simulink model "TwoTankS11_Owen_v6"  (Simulink 9.1)
settings: Solver=ode3  StartTime=0.0  StopTime=999  FixedStep=1/10  RelTol=1e-3  EnableMultiTasking=on
undefined symbols (not defined in the file or in its folder): MIO, National_Instruments, PCI
libraries: sldrtlib x3
settings Model: Creator=fowen  LastModifiedBy=melab2  SimulationMode=external  ExtModeTrigDuration=10000
settings DataIOCC: LimitDataPoints=on  MaxDataPoints=100000  SignalLoggingSaveFormat=ModelDataLogs
settings OptimizationCC: ExpressionDepthLimit=2147483647  LifeSpan=auto
settings DebuggingCC: SolverPrmCheckMsg=warning  FcnCallInpInsideContextMsg=warning  StateNameClashWarn=warning
settings HardwareCC: ProdBitPerPointer=64  ProdBitPerSizeT=64  ProdBitPerPtrDiffT=64  ProdLargestAtomicFloat=Float  ProdIntDivRoundTo=Zero  ProdEndianess=LittleEndian  ProdWordSize=64  ProdHWDeviceType=Intel->x86-64 (Windows64)
settings RTWCC: SystemTargetFile=sldrt.tlc  TemplateMakefile=sldrt.tmf  Description=Simulink Desktop Real-Time  RTWCompilerOptimization=on
settings CodeAppCC: MaxIdLength=95
settings SimulinkDesktopRealTimeCC: TargetPreCompLibLocation=C:\Program Files\MATLAB\R2018a\toolbox\sldrt\lib\win64  TargetLangStandard=C89/C90 (ANSI)  SupportVariableSizeSignals=off
settings ConfigComp: CovSFcnEnable=off

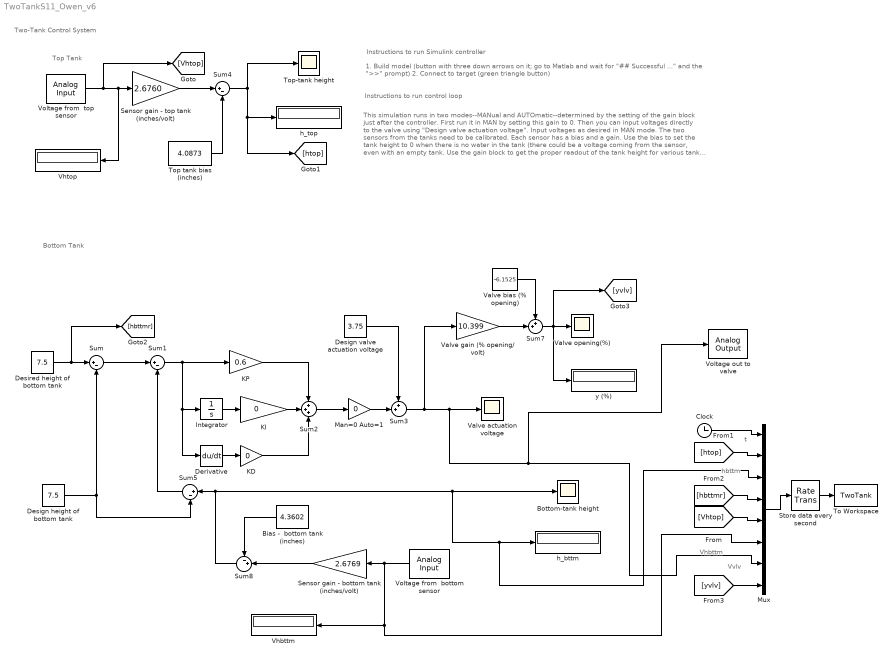
== system TwoTankS11_Owen_v6 ==
  note: Two-Tank Control System
  note: Top Tank
  note: Vhbttm
  note: Vvlv
  note: hbttm
  note: This simulation runs in two modes--MANual and AUTOmatic--determined by the setting of the gain block just after
      | the controller.  First run it in MAN by setting this gain to 0.  Then you can input voltages directly to the valve using
      | "Design valve actuation voltage".  Input voltages as desired in MAN mode.
      |
      | The two sensors from the tanks need to be calibrated.  Each sensor has a bias and a gain.  Use the bias to set the
      | tank height to 0 when there is no water in the tank (there could be a voltage coming from the sensor, even with an
      | empty tank.  Use the gain block to get the proper readout of the tank height for various tank heights.
      |
      | Likewise, the valve %-opening read-out can be calibrated.  This give a rough estimate of the valve position.  But
      | it is just working from the input voltage signal to the valve, so it should not be fully trusted.
      |
      | Once you get everything calibrated correctly and the system running at a steady state, you can run the loop in AUTO.
      | The loop works on deviations from your desired or design steady state.  Make sure that you first put the steady state
      | height of the bottom tank in "Design height of bottom tank".  Set also "Desired height of bottom tank" to this same value,
      | the beginning AND the end values.  Then the loop should run at this level until you change something.
  note: 1. Build model (button with three down arrows on it; go to Matlab and wait for "## Successful ..." and the ">>" prompt)
      | 2. Connect to target (green triangle button)
  note: Instructions to run Simulink controller
  note: Instructions to run control loop
  note: Bottom Tank
  note: t
  Bias -  bottom tank (inches) : Constant  Value=4.3602
  Bottom-tank height : Scope
  Clock : Clock
  Derivative : Derivative
  Design height of bottom tank : Constant  Value=7.5
  Design valve actuation voltage : Constant  Value=3.75
  Desired height of bottom tank : Constant  Value=7.5
  Integrator : Integrator
  KD : Gain  Gain=0
  KI : Gain  Gain=0
  KP : Gain  Gain=0.6
  Man=0 Auto=1 : Gain  Gain=0
  Mux : Mux  Inputs=8
  Sensor gain - bottom tank (inches/volt) : Gain  Gain=2.6769
  Sensor gain - top tank (inches/volt) : Gain  Gain=2.6760
  Store data every second : RateTransition  OutPortSampleTimeOpt=Inherit  OutPortSampleTimeMultiple=10  OutPortSampleTime=10
  Sum{,1,4..5} (4 alike) : Sum  Inputs=|+-
  Sum2 : Sum  Inputs=+++
  Sum3 : Sum  Inputs=++|
  Sum7 : Sum  Inputs=++|
  Sum8 : Sum  Inputs=-+|
  To Workspace : ToWorkspace  VariableName=TwoTank  SampleTime=1
  Top tank bias (inches) : Constant  Value=4.0873
  Top-tank height : Scope
  Valve actuation voltage : Scope
  Valve bias (% opening) : Constant  Value=-6.1525
  Valve gain (% opening/ volt) : Gain  Gain=10.399
  Valve opening(%) : Scope
  Vhbttm : Display
  Vhtop : Display
  Voltage from  bottom sensor : sldrtlib/Analog Input  SampleTime=1/10  MaxMissedTicks=10  ShowMissedTicks=off  YieldWhenWaiting=off  DrvName=National_Instruments/PCI-MIO-16E-4  DrvAddress=4294967295  DrvOptions=[1 0 0 0 0 0]  Channels=5  RangeMode=1  VoltRange=1  DataType=1
      settings: AttributesFormatString=National Instruments\nPCI-MIO-16E-4 [auto]  SourceProductName=Simulink Desktop Real-Time
  Voltage from  top sensor : sldrtlib/Analog Input  SampleTime=1/10  MaxMissedTicks=10  ShowMissedTicks=off  YieldWhenWaiting=off  DrvName=National_Instruments/PCI-MIO-16E-4  DrvAddress=4294967295  DrvOptions=[1 0 0 0 0 0]  Channels=4  RangeMode=1  VoltRange=1  DataType=1
      settings: AttributesFormatString=National Instruments\nPCI-MIO-16E-4 [auto]  SourceProductName=Simulink Desktop Real-Time
  Voltage out to valve : sldrtlib/Analog Output  SampleTime=1/10  MaxMissedTicks=10  ShowMissedTicks=off  YieldWhenWaiting=off  DrvName=National_Instruments/PCI-MIO-16E-4  DrvAddress=4294967295  DrvOptions=[1 0 0 0 0 0]  Channels=1  RangeMode=1  VoltRange=1  InitialValue=[]  FinalValue=[]
      settings: AttributesFormatString=National Instruments\nPCI-MIO-16E-4 [auto]  SourceProductName=Simulink Desktop Real-Time
  h_bttm : Display
  h_top : Display
  y (%) : Display
  wires:
  Desired height of bottom tank/1 -> Sum/1, [hbttmr]
  Design height of bottom tank/1 -> Sum/2, Sum5/2
  Sum/1 -> Sum1/1
  Sum1/1 -> KP/1, Integrator/1, Derivative/1
  Integrator/1 -> KI/1
  Derivative/1 -> KD/1
  KP/1 -> Sum2/1
  KI/1 -> Sum2/2
  KD/1 -> Sum2/3
  Sum3/1 -> Valve actuation voltage/1, Voltage out to valve/1, Mux/7, Valve gain (% opening/ volt)/1
  Sensor gain - bottom tank (inches/volt)/1 -> Sum8/2
  Sum8/1 -> Sum5/1, Bottom-tank height/1, h_bttm/1, Mux/3
  Sum5/1 -> Sum1/2
  Design valve actuation voltage/1 -> Sum3/1
  Sum2/1 -> Man=0 Auto=1/1
  Valve bias (% opening)/1 -> Sum7/1
  Voltage from  top sensor/1 -> [Vhtop], Sensor gain - top tank (inches/volt)/1, Vhtop/1
  Top tank bias (inches)/1 -> Sum4/2
  Sensor gain - top tank (inches/volt)/1 -> Sum4/1
  Sum4/1 -> h_top/1, [htop], Top-tank height/1
  Bias -  bottom tank (inches)/1 -> Sum8/1
  Voltage from  bottom sensor/1 -> Sensor gain - bottom tank (inches/volt)/1, Mux/6, Vhbttm/1
  Man=0 Auto=1/1 -> Sum3/2
  Mux/1 -> Store data every second/1
  Store data every second/1 -> To Workspace/1
  [Vhtop] -> Mux/5
  [hbttmr] -> Mux/4
  [htop] -> Mux/2
  Clock/1 -> Mux/1
  Sum7/1 -> [yvlv], Valve opening(%)/1, y (%)/1
  Valve gain (% opening/ volt)/1 -> Sum7/2
  [yvlv] -> Mux/8
